simulink model "p214"  (R2018b)
settings: Solver=VariableStepAuto  StartTime=0.0  StopTime=500  RelTol=1e-7
settings Model: Creator=iman  LastModifiedBy=iman

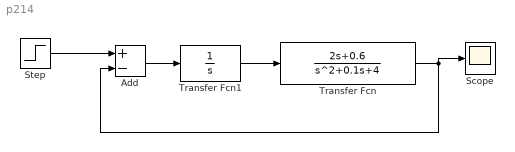
== system p214 ==
  Add : Sum  Inputs=+-
  Scope : Scope
  Step : Step  SampleTime=0
  Transfer Fcn : TransferFcn  Numerator=[ 2 0.6 ]  Denominator=[1 0.1 4 ]
  Transfer Fcn1 : TransferFcn  Denominator=[1 0]
  wires:
  Transfer Fcn1/1 -> Transfer Fcn/1
  Step/1 -> Add/1
  Add/1 -> Transfer Fcn1/1
  Transfer Fcn/1 -> Scope/1, Add/2
